simulink model "Process"  (R2022b)
settings: Solver=VariableStepAuto  StartTime=0.0  StopTime=inf  RelTol=1e-3
libraries: dspnetwork x4
settings Model: Creator=karnbongkotboonriong  LastModifiedBy=karnbongkotboonriong

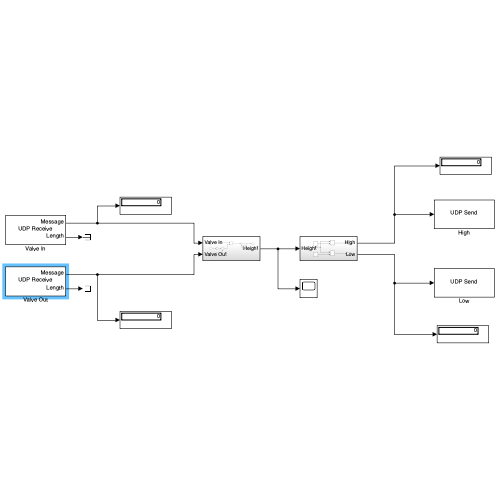
[thumbnail: Simulink's stored preview of the top-level diagram]
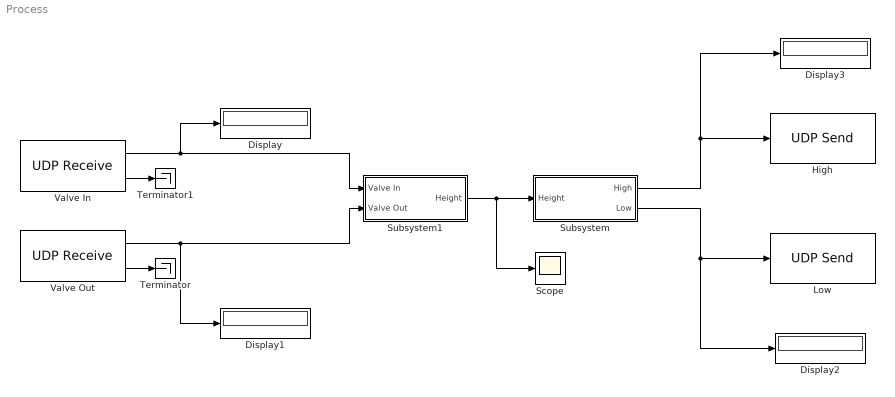
== system Process ==
  Display{,1..3} (4 alike) : Display
  High : dspnetwork/UDP Send  remoteURL='localhost'  remotePort=10001  localURL='0.0.0.0'  localPortSource=Automatically determine  localPort=-1  sendBufferSize=8192  sampletime=-1  blockPlatform=[]  separateLengthPort=0
      settings: LibrarySourceBlock=dspsnks4/UDP Send
  Low : dspnetwork/UDP Send  remoteURL='localhost'  remotePort=10002  localURL='0.0.0.0'  localPortSource=Automatically determine  localPort=-1  sendBufferSize=8192  sampletime=-1  blockPlatform=[]  separateLengthPort=0
      settings: LibrarySourceBlock=dspsnks4/UDP Send
  Scope : Scope
  Subsystem : Subsystem
  Subsystem1 : Subsystem  ScheduleAs=Aperiodic partition  PartitionName=TEMP_PRECOMP_PARTITION_NAME_MessageTriggeredSubsystem
      settings: LibrarySourceBlock=|
      | hdlsllib/Ports &
      | Subsystems/Subsystem
  Terminator : Terminator
  Terminator1 : Terminator
  Valve In : dspnetwork/UDP Receive  localURL='0.0.0.0'  localPort=10003  remoteURL='0.0.0.0'  remotePort=-1  recvBufferSize=8192  dims=1  signalDatatype=boolean  isComplex=off  isVarSize=off  showBlockingTime=off  blockingTime=0  sampletime=0.001  blockPlatform=[]
      settings: LibrarySourceBlock=dspsrcs4/UDP Receive
  Valve Out : dspnetwork/UDP Receive  localURL='0.0.0.0'  localPort=10004  remoteURL='0.0.0.0'  remotePort=-1  recvBufferSize=8192  dims=1  signalDatatype=boolean  isComplex=off  isVarSize=off  showBlockingTime=off  blockingTime=0  sampletime=0.0001  blockPlatform=[]
      settings: LibrarySourceBlock=dspsrcs4/UDP Receive
  wires:
  Subsystem/1(High) -> Display3/1, High/1
  Subsystem/2(Low) -> Display2/1, Low/1
  Subsystem1/1(Height) -> Scope/1, Subsystem/1(Height)
  Valve In/2 -> Terminator1/1
  Valve Out/2 -> Terminator/1
  Valve Out/1 -> Subsystem1/2(Valve Out), Display1/1
  Valve In/1 -> Subsystem1/1(Valve In), Display/1

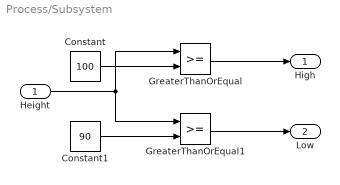
== system Process/Subsystem ==
  Height : Inport
  Constant : Constant  Value=100
  Constant1 : Constant  Value=90
  GreaterThanOrEqual : RelationalOperator  OutDataTypeStr=boolean  RndMeth=Simplest  InputSameDT=off
  GreaterThanOrEqual1 : RelationalOperator  OutDataTypeStr=boolean  RndMeth=Simplest  InputSameDT=off
  High : Outport
  Low : Outport  Port=2
  wires:
  GreaterThanOrEqual/1 -> High/1
  GreaterThanOrEqual1/1 -> Low/1
  Height/1 -> GreaterThanOrEqual1/1, GreaterThanOrEqual/1
  Constant1/1 -> GreaterThanOrEqual1/2
  Constant/1 -> GreaterThanOrEqual/2

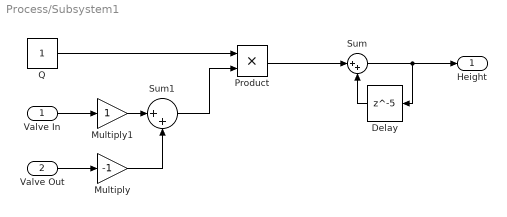
== system Process/Subsystem1 ==
  Valve In : Inport
  Valve Out : Inport  Port=2
  Delay : Delay  DelayLength=5
  Multiply : Gain  Gain=-1
  Multiply1 : Gain
  Product : Product
  Q : Constant
  Sum : Sum  Inputs=|++
  Sum1 : Sum  Inputs=|++
  Height : Outport
  wires:
  Q/1 -> Product/1
  Multiply1/1 -> Sum1/1
  Sum1/1 -> Product/2
  Product/1 -> Sum/1
  Multiply/1 -> Sum1/2
  Sum/1 -> Delay/1, Height/1
  Valve In/1 -> Multiply1/1
  Valve Out/1 -> Multiply/1
  Delay/1 -> Sum/2
